simulink model "car_kine3"  (R2019a)
settings: Solver=VariableStepAuto  StartTime=0.0  StopTime=20.0  RelTol=1e-3
libraries: simulink x1
settings Model: Creator=mi  LastModifiedBy=mi

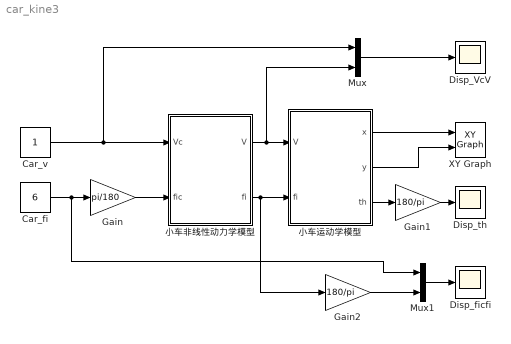
== system car_kine3 ==
  Car_fi : Constant  Value=6
  Car_v : Constant
  "Disp_VcV " : Scope
  "Disp_ficfi " : Scope
  "Disp_th " : Scope
  Gain : Gain  Gain=pi/180
  Gain1 : Gain  Gain=180/pi
  Gain2 : Gain  Gain=180/pi
  Mux : Mux  Inputs=2
  Mux1 : Mux  Inputs=2
  XY Graph : simulink/Sinks/XY Graph  xmin=-3  xmax=3  ymin=-0.2  ymax=5.2  st=-1
  "小车运动学模型 " : Subsystem  mask{L=0.254}
      mask prompts: L "小车车长L(米)"
  小车非线性动力学模型 : Subsystem  mask{M=1.4175, L=0.254, W=6.5*2.54/100, bu=14.175, b=3.5*2.54/100, Tv=0.1, Tfi=0.1}
      mask prompts: M "小车质量(千克)"; L "车长(米)"; W "车宽(米)"; bu "小车前向阻尼系数"; b "小车质心到后轮的距离(米)"; Tv "小车速度驱动时间常数(秒)"; Tfi "小车转向驱动时间常数(秒)"
      mask init:
      | J=M*(L^2+W^2)/12
  wires:
  "小车运动学模型 "/3("th ") -> Gain1/1
  Gain1/1 -> "Disp_th "/1
  "小车运动学模型 "/1(x) -> XY Graph/1
  "小车运动学模型 "/2(y) -> XY Graph/2
  Car_fi/1 -> Mux1/1, Gain/1
  Gain/1 -> 小车非线性动力学模型/2(fic)
  小车非线性动力学模型/1(V) -> Mux/2, "小车运动学模型 "/1(V)
  小车非线性动力学模型/2("fi ") -> Gain2/1, "小车运动学模型 "/2(fi)
  Car_v/1 -> Mux/1, 小车非线性动力学模型/1(Vc)
  Mux/1 -> "Disp_VcV "/1
  Mux1/1 -> "Disp_ficfi "/1
  Gain2/1 -> Mux1/2

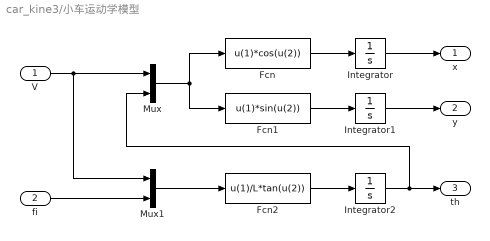
== system car_kine3/小车运动学模型  ==
  V : Inport
  fi : Inport  Port=2
  Fcn : Fcn  Expr=u(1)*cos(u(2))
  Fcn1 : Fcn  Expr=u(1)*sin(u(2))
  Fcn2 : Fcn  Expr=u(1)/L*tan(u(2))
  Integrator : Integrator
  Integrator1 : Integrator
  Integrator2 : Integrator
  Mux : Mux  Inputs=2
  Mux1 : Mux  Inputs=2
  x : Outport
  y : Outport  Port=2
  "th " : Outport  Port=3
  wires:
  Integrator2/1 -> "th "/1, Mux/2
  Fcn/1 -> Integrator/1
  Mux1/1 -> Fcn2/1
  Fcn2/1 -> Integrator2/1
  fi/1 -> Mux1/2
  Integrator1/1 -> y/1
  Mux/1 -> Fcn/1, Fcn1/1
  V/1 -> Mux1/1, Mux/1
  Integrator/1 -> x/1
  Fcn1/1 -> Integrator1/1

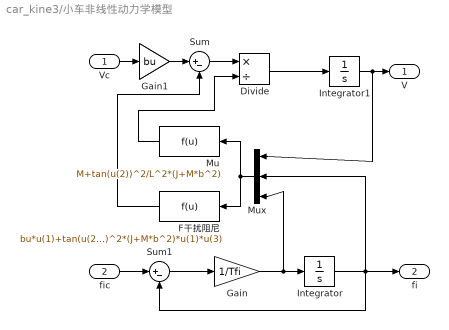
== system car_kine3/小车非线性动力学模型 ==
  Vc : Inport
  fic : Inport  Port=2
  Divide : Product  Inputs=*/
  F干扰阻尼 : Fcn  Expr=bu*u(1)+tan(u(2))/L^2/cos(u(2))^2*(J+M*b^2)*u(1)*u(3)
  Gain : Gain  Gain=1/Tfi
  Gain1 : Gain  Gain=bu
  Integrator : Integrator
  Integrator1 : Integrator
  Mu : Fcn  Expr=M+tan(u(2))^2/L^2*(J+M*b^2)
  Mux : Mux  Inputs=3
  Sum : Sum  Inputs=|+-
  Sum1 : Sum  Inputs=|+-
  V : Outport
  "fi " : Outport  Port=2
  wires:
  fic/1 -> Sum1/1
  Sum1/1 -> Gain/1
  Gain/1 -> Mux/3, Integrator/1
  Integrator/1 -> Mux/2, Sum1/2, "fi "/1
  Integrator1/1 -> Mux/1, V/1
  Divide/1 -> Integrator1/1
  Sum/1 -> Divide/1
  Mux/1 -> F干扰阻尼/1, Mu/1
  Mu/1 -> Divide/2
  F干扰阻尼/1 -> Sum/2
  Vc/1 -> Gain1/1
  Gain1/1 -> Sum/1
